simulink model "examination_Ver_2"  (R2015b)
settings: Solver=VariableStepAuto  StartTime=0.0  StopTime=inf  RelTol=1e-3
libraries: robotlib x12
settings Model: Creator=weberhsu  LastModifiedBy=weberhsu

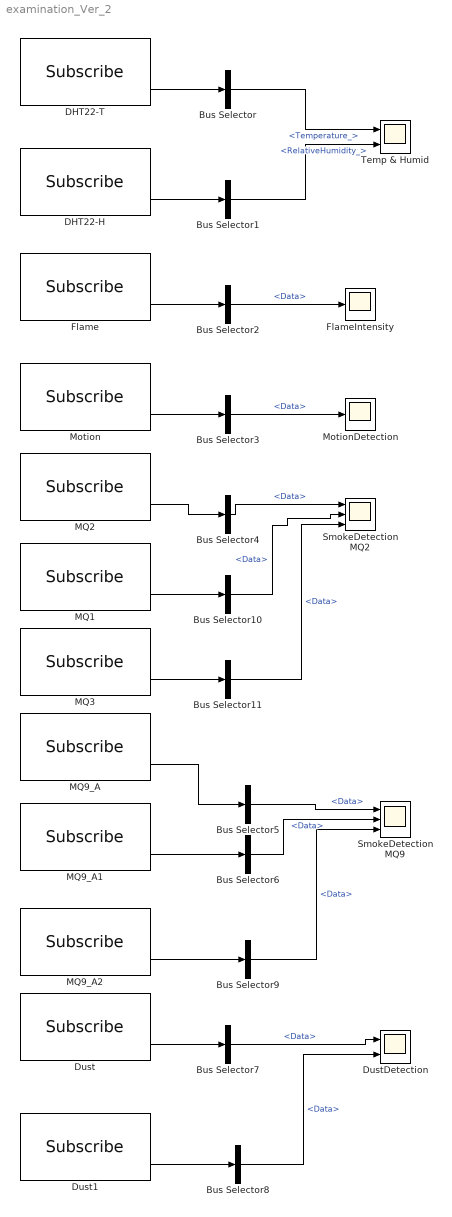
== system examination_Ver_2 ==
  Bus Selector : BusSelector  OutputSignals=Temperature_
  Bus Selector1 : BusSelector  OutputSignals=RelativeHumidity_
  Bus Selector{2..11} (10 alike) : BusSelector  OutputSignals=Data
  DHT22-H : robotlib/Subscribe  SourceLibraryInfo=This block requires Robotics System Toolbox  topicSource=Select from ROS network  topic=/CurHumidity  messageType=sensor_msgs/RelativeHumidity  sampleTime=-1  messageQueueLength=1
  DHT22-T : robotlib/Subscribe  SourceLibraryInfo=This block requires Robotics System Toolbox  topicSource=Select from ROS network  topic=/CurTemperature  messageType=sensor_msgs/Temperature  sampleTime=-1  messageQueueLength=1
  Dust : robotlib/Subscribe  SourceLibraryInfo=This block requires Robotics System Toolbox  topicSource=Select from ROS network  topic=/DustDetection  messageType=std_msgs/Float32  sampleTime=-1  messageQueueLength=1
  Dust1 : robotlib/Subscribe  SourceLibraryInfo=This block requires Robotics System Toolbox  topicSource=Select from ROS network  topic=/DustDetectionV  messageType=std_msgs/Float32  sampleTime=-1  messageQueueLength=1
  DustDetection : Scope  NumInputPorts=2
  Flame : robotlib/Subscribe  SourceLibraryInfo=This block requires Robotics System Toolbox  topicSource=Select from ROS network  topic=/FlameDetection  messageType=std_msgs/Float32  sampleTime=-1  messageQueueLength=1
  FlameIntensity : Scope
  MQ1 : robotlib/Subscribe  SourceLibraryInfo=This block requires Robotics System Toolbox  topicSource=Select from ROS network  topic=/MQ2LPG  messageType=std_msgs/Float32  sampleTime=-1  messageQueueLength=1
  MQ2 : robotlib/Subscribe  SourceLibraryInfo=This block requires Robotics System Toolbox  topicSource=Select from ROS network  topic=/MQ2CO  messageType=std_msgs/Float32  sampleTime=-1  messageQueueLength=1
  MQ3 : robotlib/Subscribe  SourceLibraryInfo=This block requires Robotics System Toolbox  topicSource=Select from ROS network  topic=/MQ2SMOKE  messageType=std_msgs/Float32  sampleTime=-1  messageQueueLength=1
  MQ9_A : robotlib/Subscribe  SourceLibraryInfo=This block requires Robotics System Toolbox  topicSource=Select from ROS network  topic=/MQ9LPG  messageType=std_msgs/Float32  sampleTime=-1  messageQueueLength=1
  MQ9_A1 : robotlib/Subscribe  SourceLibraryInfo=This block requires Robotics System Toolbox  topicSource=Select from ROS network  topic=/MQ9CO  messageType=std_msgs/Float32  sampleTime=-1  messageQueueLength=1
  MQ9_A2 : robotlib/Subscribe  SourceLibraryInfo=This block requires Robotics System Toolbox  topicSource=Select from ROS network  topic=/MQ9CH4  messageType=std_msgs/Float32  sampleTime=-1  messageQueueLength=1
  Motion : robotlib/Subscribe  SourceLibraryInfo=This block requires Robotics System Toolbox  topicSource=Select from ROS network  topic=/MotionDetection  messageType=std_msgs/Bool  sampleTime=-1  messageQueueLength=1
  MotionDetection : Scope
  SmokeDetection MQ2 : Scope  NumInputPorts=3
  SmokeDetection MQ9 : Scope  NumInputPorts=3
  Temp & Humid : Scope  NumInputPorts=2
  wires:
  DHT22-T/2 -> Bus Selector/1
  Bus Selector/1 -> Temp & Humid/1  "<Temperature_>"
  DHT22-H/2 -> Bus Selector1/1
  Bus Selector1/1 -> Temp & Humid/2  "<RelativeHumidity_>"
  Flame/2 -> Bus Selector2/1
  Bus Selector2/1 -> FlameIntensity/1  "<Data>"
  Motion/2 -> Bus Selector3/1
  Bus Selector3/1 -> MotionDetection/1  "<Data>"
  MQ2/2 -> Bus Selector4/1
  Bus Selector4/1 -> SmokeDetection MQ2/1  "<Data>"
  MQ9_A/2 -> Bus Selector5/1
  Bus Selector5/1 -> SmokeDetection MQ9/1  "<Data>"
  Dust/2 -> Bus Selector7/1
  Bus Selector7/1 -> DustDetection/1  "<Data>"
  Dust1/2 -> Bus Selector8/1
  Bus Selector8/1 -> DustDetection/2  "<Data>"
  MQ9_A1/2 -> Bus Selector6/1
  MQ9_A2/2 -> Bus Selector9/1
  Bus Selector6/1 -> SmokeDetection MQ9/2  "<Data>"
  Bus Selector9/1 -> SmokeDetection MQ9/3  "<Data>"
  MQ1/2 -> Bus Selector10/1
  MQ3/2 -> Bus Selector11/1
  Bus Selector10/1 -> SmokeDetection MQ2/2  "<Data>"
  Bus Selector11/1 -> SmokeDetection MQ2/3  "<Data>"
